simulink model "fmcw_simu"  (R2025b)
settings: Solver=FixedStepDiscrete  StartTime=0.0  StopTime=2e-3  FixedStep=1/40e6  RelTol=1e-3
undefined symbols (not defined in the file or in its folder): physconst, tgt_pos, tx_pos, vel_zero
libraries: phasedenvlib x3, phaseddetectlib x1, dspxfrm3 x1, phasedwavlib x1
settings Model: Creator=mehme  LastModifiedBy=mehme

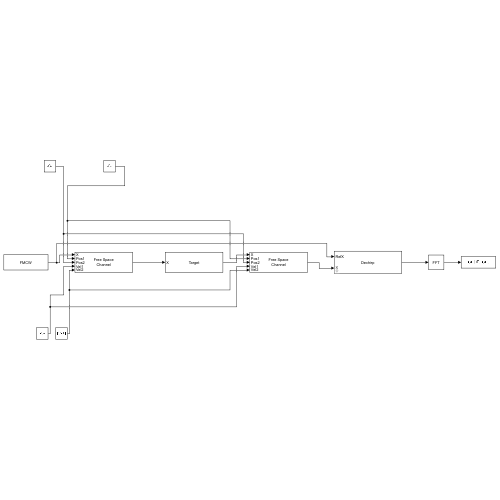
[thumbnail: Simulink's stored preview of the top-level diagram]
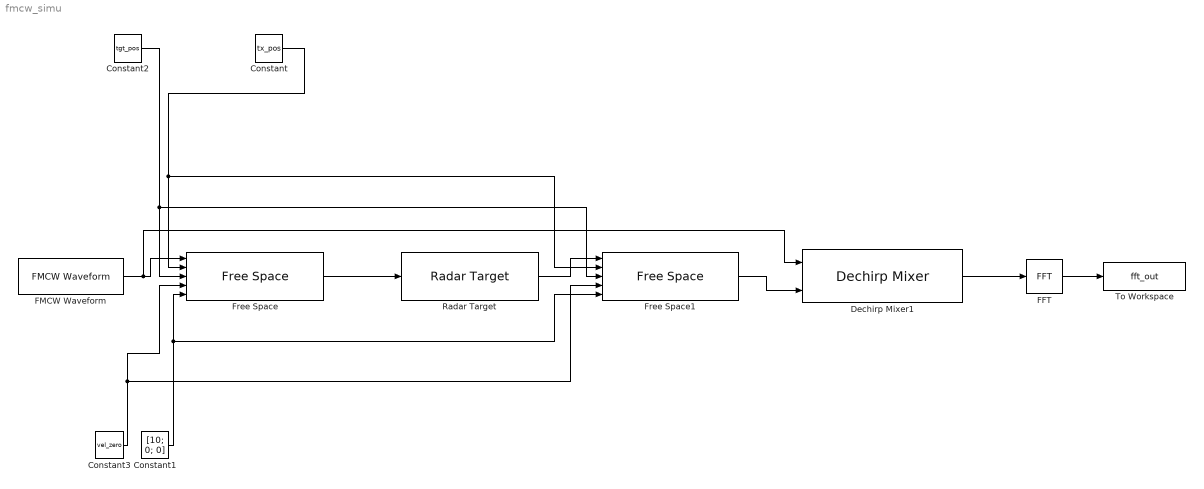
== system fmcw_simu ==
  Constant : Constant  Value=tx_pos  VectorParams1D=off
  Constant1 : Constant  Value=[10; 0; 0]  VectorParams1D=off
  Constant2 : Constant  Value=tgt_pos  VectorParams1D=off
  Constant3 : Constant  Value=vel_zero  VectorParams1D=off
  Dechirp Mixer1 : phaseddetectlib/Dechirp Mixer
  FFT : dspxfrm3/FFT  FFTImplementation=Auto  CompMethod=Table lookup  TableOpt=NEW  TableOptActive=Speed  BitRevOrder=off  Normalize=off  InheritFFTLength=on  FFTLength=64  WrapInput=on  roundingMode=Ceiling  overflowMode=off  firstCoeffDataTypeStr=Inherit: Same word length as input  firstCoeffLastDataTypeStr=Inherit: Same word length as input  outputMin=[]  outputMax=[]
  FMCW Waveform : phasedwavlib/FMCW Waveform  SampleRate=fs  SweepTime=T  SweepBandwidth=B  SweepDirection=Up  SweepInterval=Positive  OutputFormat=Sweeps  NumSamples=100  NumSweeps=1  SimulateUsing=Interpreted execution
  Free Space : phasedenvlib/Free Space  PropagationSpeed=physconst( 'LightSpeed' )  OperatingFrequency=f0  TwoWayPropagation=off  SampleRateFromInputCheckbox=on  SampleRate=1e6  MaximumDistanceSource=Property  MaximumDistance=500  MaximumNumInputSamplesSource=Auto  MaximumNumInputSamples=1000  SimulateUsing=Interpreted execution
  Free Space1 : phasedenvlib/Free Space  PropagationSpeed=physconst( 'LightSpeed' )  OperatingFrequency=f0  TwoWayPropagation=off  SampleRateFromInputCheckbox=on  SampleRate=1e6  MaximumDistanceSource=Property  MaximumDistance=500  MaximumNumInputSamplesSource=Auto  MaximumNumInputSamples=1000  SimulateUsing=Interpreted execution
  Radar Target : phasedenvlib/Radar Target  EnablePolarization=off  Mode=Monostatic  MeanRCSSource=Property  ScatteringMatrixSource=Property  MeanRCS=1  ScatteringMatrix=eye( 2 )  Model=Nonfluctuating  PropagationSpeed=physconst( 'LightSpeed' )  OperatingFrequency=2.4e9  SeedSource=Auto  Seed=0  SimulateUsing=Interpreted execution
  To Workspace : ToWorkspace  VariableName=fft_out  SampleTime=-1
  wires:
  FMCW Waveform/1 -> Dechirp Mixer1/1, Free Space/1
  Free Space/1 -> Radar Target/1
  Radar Target/1 -> Free Space1/1
  Free Space1/1 -> Dechirp Mixer1/2
  Dechirp Mixer1/1 -> FFT/1
  Constant/1 -> Free Space1/2, Free Space/2
  Constant2/1 -> Free Space1/3, Free Space/3
  Constant3/1 -> Free Space1/4, Free Space/4
  Constant1/1 -> Free Space1/5, Free Space/5
  FFT/1 -> To Workspace/1
